simulink model "Optitrack_get"  (R2015a)
settings: Solver=ode45  StartTime=0.0  StopTime=inf  RelTol=1e-3
libraries: robotlib x1
settings Model: Creator=rshu  LastModifiedBy=rshu

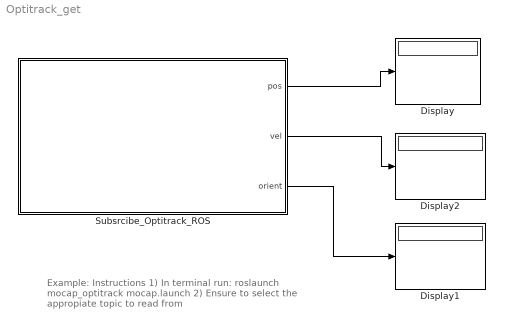
== system Optitrack_get ==
  note: Example:
      |
      | Instructions
      | 1) In terminal run:
      | roslaunch mocap_optitrack mocap.launch
      | 2) Ensure to select the appropiate topic to read from
  Display : Display
  Display1 : Display
  Display2 : Display
  Subsrcibe_Optitrack_ROS : Subsystem
      mask Display:
      | image('prime41-optitrack.png');
      | color('cyan')
      | port_label('output',1,'pos [vector]');
      | port_label('output',2,'vel [vector]');
      | port_label('output',3,'orient [euler]');
  wires:
  Subsrcibe_Optitrack_ROS/1(pos) -> Display/1
  Subsrcibe_Optitrack_ROS/3(orient) -> Display1/1
  Subsrcibe_Optitrack_ROS/2(vel) -> Display2/1

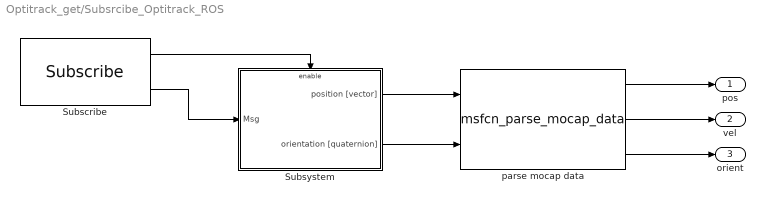
== system Optitrack_get/Subsrcibe_Optitrack_ROS ==
  Subscribe : robotlib/Subscribe  SourceLibraryInfo=This block requires Robotics System Toolbox  topicSource=Select from ROS network  topic=/CF/pose  messageType=geometry_msgs/PoseStamped  sampleTime=-1  messageQueueLength=1
  Subsystem : Subsystem
  parse mocap data : M-S-Function  FunctionName=msfcn_parse_mocap_data
      mask Display:
      | port_label('input', 1, 'pos')
      | port_label('input', 2, 'ornt')
      | 
      | port_label('output', 1, 'pos')
      | port_label('output', 2, 'vel')
      | port_label('output', 3, 'ornt [Euler]')
  pos : Outport
  vel : Outport  Port=2
  orient : Outport  Port=3
  wires:
  Subsystem/1(position [vector]) -> parse mocap data/1
  Subscribe/2 -> Subsystem/1(Msg)
  Subscribe/1 -> Subsystem/Enable
  parse mocap data/3 -> orient/1
  parse mocap data/2 -> vel/1
  Subsystem/2(orientation [quaternion]) -> parse mocap data/2
  parse mocap data/1 -> pos/1

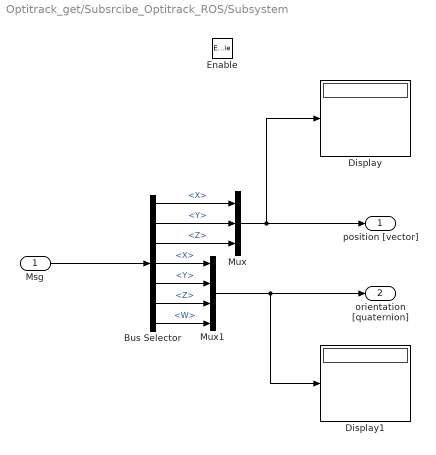
== system Optitrack_get/Subsrcibe_Optitrack_ROS/Subsystem ==
  Msg : Inport
  Enable : EnablePort
  Bus Selector : BusSelector  OutputSignals=Pose.Position.X,Pose.Position.Y,Pose.Position.Z,Pose.Orientation.X,Pose.Orientation.Y,Pose.Orientation.Z,Pose.Orientation.W
  Display : Display
  Display1 : Display
  Mux : Mux  Inputs=3
  Mux1 : Mux
  position [vector] : Outport
  orientation [quaternion] : Outport  Port=2
  wires:
  Msg/1 -> Bus Selector/1
  Bus Selector/1 -> Mux/1  "<X>"
  Bus Selector/2 -> Mux/2  "<Y>"
  Bus Selector/3 -> Mux/3  "<Z>"
  Mux/1 -> position [vector]/1, Display/1
  Bus Selector/4 -> Mux1/1  "<X>"
  Bus Selector/5 -> Mux1/2  "<Y>"
  Bus Selector/6 -> Mux1/3  "<Z>"
  Bus Selector/7 -> Mux1/4  "<W>"
  Mux1/1 -> Display1/1, orientation [quaternion]/1
